simulink model "untitled23"  (R2019a)
settings: Solver=VariableStepAuto  StartTime=0.0  StopTime=10.0  RelTol=1e-3
values from neighbouring files (symbols this model uses):
  a0 = 3    [Gradient_instant_cost.m]    (also in Gradient_integral_cost.m; MRAC.m = 3+n(1); MRAC2.m = 1+n(1); MRAC3.m = 1)
  am = 1    [Untitled34.m]
  b0 = 1    [Gradient_instant_cost.m]    (also in Gradient_integral_cost.m; MRAC.m = 7+n(3); MRAC2.m = 3+n(3); MRAC3.m = 3)
  gamma = diag([0.01,0.01,0.005,0.005])    [MRAC3.m]    (also in Parameter_estimation.m = 10*i; Untitled2.m = 10; Untitled34.m = 1; Untitled9.m = 1)
settings Model: Creator=Student  LastModifiedBy=Student

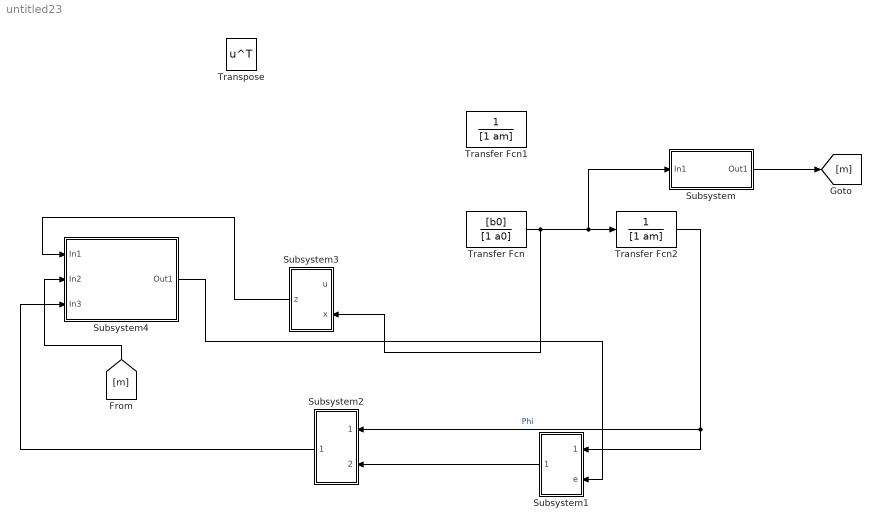
== system untitled23 ==
  Subsystem : Subsystem
  Subsystem1 : Subsystem
  Subsystem2 : Subsystem
  Subsystem3 : Subsystem
  Subsystem4 : Subsystem
  Transfer Fcn : TransferFcn  Numerator=[b0]  Denominator=[1 a0]
  Transfer Fcn1 : TransferFcn  Denominator=[1 am]
  Transfer Fcn2 : TransferFcn  Denominator=[1 am]
  Transpose : Math  Operator=transpose  SaturateOnIntegerOverflow=on
  wires:
  Subsystem/1(Out1) -> [m]
  ? -> Transfer Fcn/1, Subsystem3/1(u)
  Transfer Fcn/1 -> Subsystem3/2(x), Subsystem/1(In1), Transfer Fcn2/1
  Transfer Fcn2/1 -> Subsystem2/1(phi), Subsystem1/1(Phi)  "Phi"
  Subsystem1/1("theta ") -> Subsystem2/2(theta)
  Subsystem3/1(z) -> Subsystem4/1(In1)
  [m] -> Subsystem4/2(In2)
  Subsystem2/1(zhat) -> Subsystem4/3(In3)
  Subsystem4/1(Out1) -> Subsystem1/2("e ")

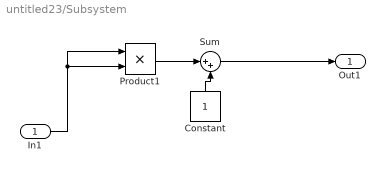
== system untitled23/Subsystem ==
  In1 : Inport
  Constant : Constant
  Product1 : Product
  Sum : Sum  Inputs=|++
  Out1 : Outport
  wires:
  Constant/1 -> Sum/2
  In1/1 -> Product1/1, Product1/2
  Sum/1 -> Out1/1
  Product1/1 -> Sum/1

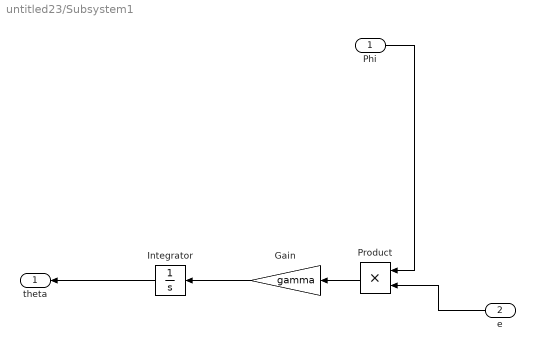
== system untitled23/Subsystem1 ==
  Phi : Inport
  "e " : Inport  Port=2
  Gain : Gain  Gain=gamma
  Integrator : Integrator
  Product : Product
  "theta " : Outport
  wires:
  Gain/1 -> Integrator/1
  Integrator/1 -> "theta "/1
  "e "/1 -> Product/2
  Product/1 -> Gain/1
  Phi/1 -> Product/1

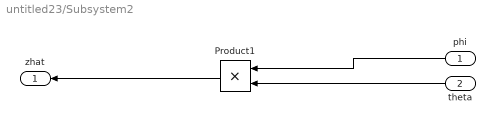
== system untitled23/Subsystem2 ==
  phi : Inport
  theta : Inport  Port=2
  Product1 : Product
  zhat : Outport
  wires:
  Product1/1 -> zhat/1
  theta/1 -> Product1/2
  phi/1 -> Product1/1

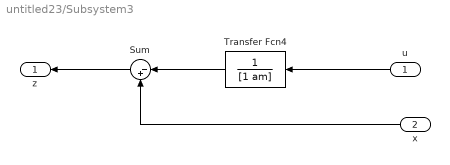
== system untitled23/Subsystem3 ==
  u : Inport
  x : Inport  Port=2
  Sum : Sum  Inputs=|-+
  Transfer Fcn4 : TransferFcn  Denominator=[1 am]
  z : Outport
  wires:
  Transfer Fcn4/1 -> Sum/1
  Sum/1 -> z/1
  u/1 -> Transfer Fcn4/1
  x/1 -> Sum/2

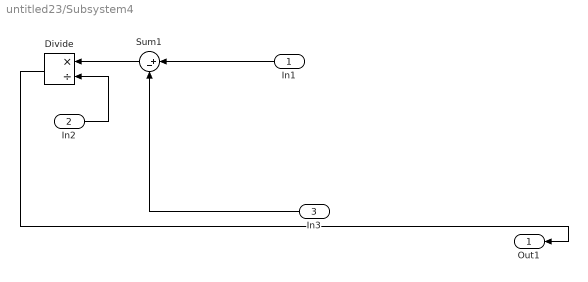
== system untitled23/Subsystem4 ==
  In1 : Inport
  In2 : Inport  Port=2
  In3 : Inport  Port=3
  Divide : Product  Inputs=*/
  Sum1 : Sum  Inputs=|+-
  Out1 : Outport
  wires:
  In3/1 -> Sum1/2
  Sum1/1 -> Divide/1
  In2/1 -> Divide/2
  In1/1 -> Sum1/1
  Divide/1 -> Out1/1
